simulink model "lqr_linearized_system"  (R2021b)
settings: Solver=VariableStepAuto  StartTime=0.0  StopTime=10  RelTol=1e-3
values from neighbouring files (symbols this model uses):
  A = [     0 0 0 1 0 0 0 0 0 0 0 0 ... (first row only)    [model_equations.m]
  Ad = sys_dt.A    [discretization.m]    (also in dlqr_kalman_controller.m; pole_placement.m)
  B = [ ... (first row only)    [model_equations.m]
  Bd = sys_dt.B    [discretization.m]    (also in dlqr_kalman_controller.m; pole_placement.m)
  K = G*inv(X)    [pole_placement.m]
settings Model: Creator=viking  LastModifiedBy=viking

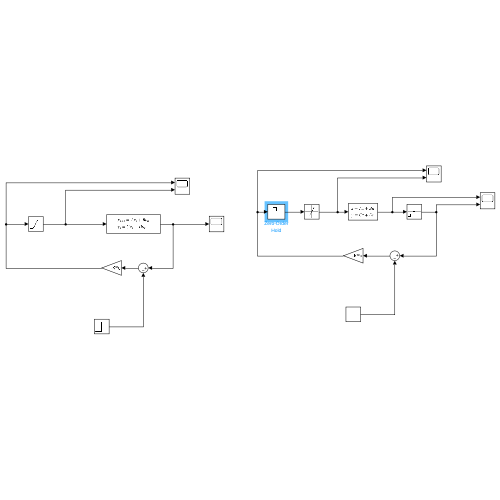
[thumbnail: Simulink's stored preview of the top-level diagram]
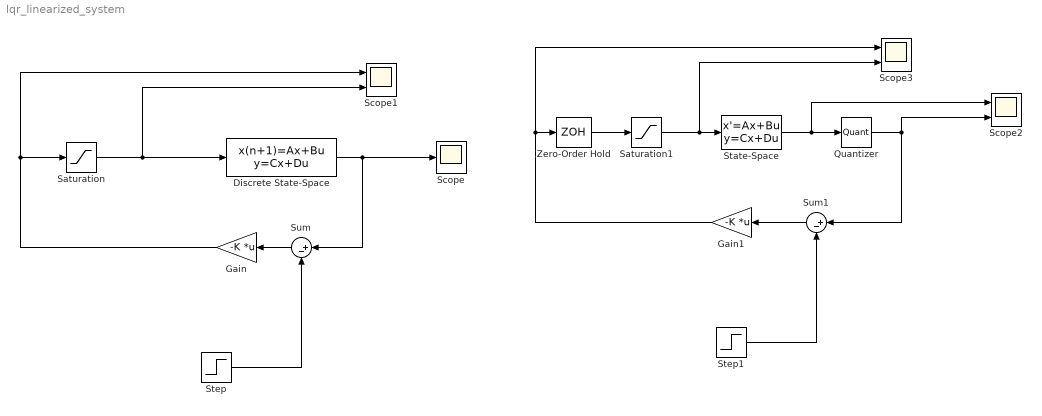
== system lqr_linearized_system ==
  Discrete State-Space : DiscreteStateSpace  A=Ad  B=Bd  C=eye(12, 12)  D=zeros(12, 4)  SampleTime=0.05
  Gain : Gain  Gain=-K  Multiplication=Matrix(K*u)
  Gain1 : Gain  Gain=-K  Multiplication=Matrix(K*u)
  Quantizer : Quantizer  QuantizationInterval=0.05
  Saturation : Saturate  UpperLimit=100  LowerLimit=0
  Saturation1 : Saturate  UpperLimit=100  LowerLimit=0
  Scope : Scope
  Scope1 : Scope  NumInputPorts=2
  Scope2 : Scope  NumInputPorts=2
  Scope3 : Scope  NumInputPorts=2
  State-Space : StateSpace  A=A  B=B  C=eye(12, 12)  D=zeros(12, 4)  InitialCondition=0
  Step : Step  Before=[0, 0, 0, 0, 0, 0, 0, 0, 0, 0, 0, 0]  After=[1, 1, 1, 0, 0, 0, 0, 0, 0, 0, 0, 0]  SampleTime=0
  Step1 : Step  Before=[0, 0, 0, 0, 0, 0, 0, 0, 0, 0, 0, 0]  After=[1, 1, 1, 0, 0, 0, 0, 0, 0, 0, 0, 0]  SampleTime=0
  Sum : Sum  Inputs=|+-
  Sum1 : Sum  Inputs=|+-
  Zero-Order Hold : ZeroOrderHold  SampleTime=0.05
  wires:
  Discrete State-Space/1 -> Sum/1, Scope/1
  Gain/1 -> Scope1/1, Saturation/1
  Sum/1 -> Gain/1
  Step/1 -> Sum/2
  Saturation/1 -> Scope1/2, Discrete State-Space/1
  Quantizer/1 -> Sum1/1, Scope2/2
  Gain1/1 -> Scope3/1, Zero-Order Hold/1
  Sum1/1 -> Gain1/1
  Step1/1 -> Sum1/2
  State-Space/1 -> Scope2/1, Quantizer/1
  Saturation1/1 -> Scope3/2, State-Space/1
  Zero-Order Hold/1 -> Saturation1/1
